simulink model "sampleModel1987"  (R2023a)
settings: Solver=VariableStepAuto  StartTime=0.0  StopTime=10.0  RelTol=1e-3
libraries: hdlsllib x4, simulink x3
settings Model: Creator=user1  LastModifiedBy=user1

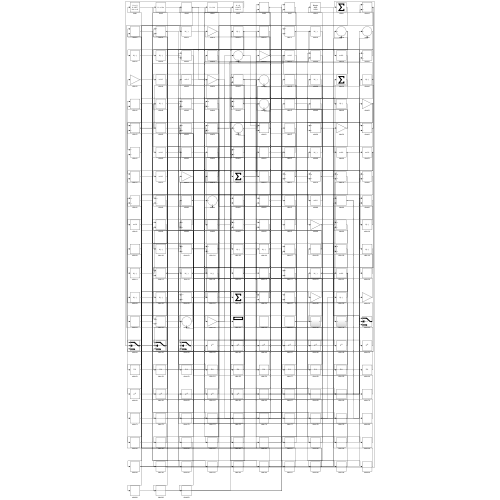
[thumbnail: Simulink's stored preview of the top-level diagram]
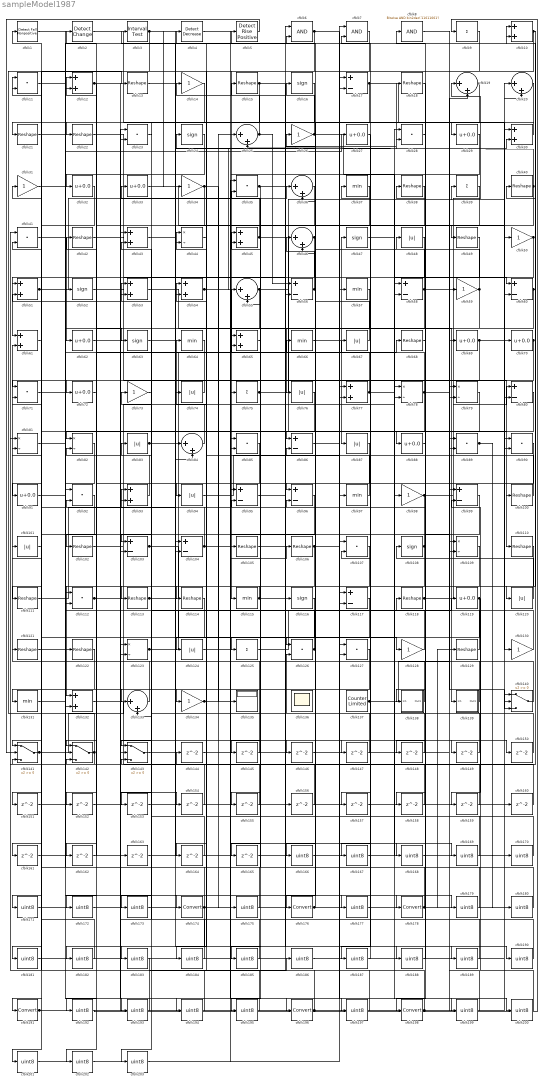
== system sampleModel1987 ==
  cfblk1 : hdlsllib/Logic and Bit Operations/Detect Fall Nonpositive  vinit=0  OutDataTypeStr=boolean
  cfblk{10,12,30,43,45,51,53..54,61,65,77,93,132} (13 alike) : Sum
  cfblk{13,15,18,21..22,38,40,42,49,68,100,102,105..106,110..111,113..114,118,121..122,129} (22 alike) : Reshape
  cfblk{48,67,74,76,83,87,94,101,120,124} (10 alike) : Abs  SaturateOnIntegerOverflow=off
  cfblk{17,56,58,60,80,86,95..96,99,103..104,117} (12 alike) : Sum  Inputs=+-
  cfblk{11,23,28,35,41,71,85,89..90,92,107,112,126..127} (14 alike) : DotProduct  OutDataTypeStr=Inherit: Inherit via internal rule
  cfblk{16,24,47,52,63,108,116} (7 alike) : Signum
  cfblk{44,78..79,81..82,109,123} (7 alike) : Product  Inputs=*/  RndMeth=Zero  SaturateOnIntegerOverflow=on
  cfblk{37,57,64,66,97,115,131} (7 alike) : MinMax
  cfblk{27,29,32..33,62,69..70,72,88,91,119} (11 alike) : Bias  Bias=0.0  SaturateOnIntegerOverflow=off
  cfblk{9,39,75,125} (4 alike) : Sum  Inputs=+
  cfblk{14,26,31,34,50,59,73,98,128,130,134} (11 alike) : Gain
  cfblk{19..20,25,36,46,55,84,133} (8 alike) : Sum  Inputs=|++
  cfblk135 : Display
  cfblk136 : Scope
      settings: Floating=on
  cfblk137 : hdlsllib/Sources/Counter Limited  uplimit=7  tsamp=-1
  cfblk138 : Subsystem
      settings: LibrarySourceBlock=|
      | hdlsllib/Ports &
      | Subsystems/Subsystem
  cfblk139 : Subsystem
      settings: LibrarySourceBlock=|
      | hdlsllib/Ports &
      | Subsystems/Subsystem
  cfblk{140..143} (4 alike) : Switch  SaturateOnIntegerOverflow=off  InputSameDT=off
  cfblk{144..165} (22 alike) : Delay  SampleTime=1
  cfblk{166..173,175,177,179..190,192..195,197,199..203} (32 alike) : DataTypeConversion  OutDataTypeStr=uint8  SaturateOnIntegerOverflow=off  RndMeth=Floor
  cfblk{174,176,178,191,196,198} (6 alike) : DataTypeConversion  SaturateOnIntegerOverflow=off  RndMeth=Floor
  cfblk2 : simulink/Logic and Bit Operations/Detect Change  vinit=0  OutDataTypeStr=boolean
      settings: LibrarySourceBlock=|
      | hdlsllib/Logic and Bit
      | Operations/Detect
      | Change
  cfblk3 : hdlsllib/Logic and Bit Operations/Interval Test  IntervalClosedRight=on  uplimit=0.5  IntervalClosedLeft=on  lowlimit=-0.5  OutDataTypeStr=boolean
  cfblk4 : simulink/Logic and Bit Operations/Detect Decrease  vinit=0.0  OutDataTypeStr=boolean
      settings: LibrarySourceBlock=|
      | hdlsllib/Logic and Bit
      | Operations/Detect
      | Decrease
  cfblk5 : hdlsllib/Logic and Bit Operations/Detect Rise Positive  vinit=0  OutDataTypeStr=boolean
  cfblk6 : Logic  AllPortsSameDT=off  OutDataTypeStr=boolean
  cfblk7 : Logic  AllPortsSameDT=off  OutDataTypeStr=boolean
  cfblk8 : simulink/Logic and Bit Operations/Bitwise Operator  logicop=AND  UseBitMask=on  BitMask=bin2dec('11011001')  BitMaskRealWorld=Stored Integer
      settings: LibrarySourceBlock=|
      | hdlsllib/Logic and Bit
      | Operations/Bitwise
      | Operator
  wires:
  cfblk16/1 -> cfblk21/1
  cfblk17/1 -> cfblk29/1, cfblk46/2
  cfblk29/1 -> cfblk115/1
  cfblk54/1 -> cfblk18/1, cfblk149/1
  cfblk77/1 -> cfblk47/1, cfblk189/1
  cfblk46/1 -> cfblk61/1, cfblk65/2
  cfblk84/1 -> cfblk64/1
  cfblk118/1 -> cfblk19/1, cfblk140/3
  cfblk133/1 -> cfblk61/2
  cfblk61/1 -> cfblk11/1
  cfblk63/1 -> cfblk86/1
  cfblk66/1 -> cfblk87/1
  cfblk100/1 -> cfblk54/1
  cfblk7/1 -> cfblk75/1
  cfblk113/1 -> cfblk55/1, cfblk147/1
  cfblk51/1 -> cfblk36/1, cfblk27/1
  cfblk132/1 -> cfblk40/1
  cfblk35/1 -> cfblk125/1, cfblk79/2, cfblk190/1
  cfblk30/1 -> cfblk22/1
  cfblk86/1 -> cfblk97/1
  cfblk95/1 -> cfblk178/1
  cfblk121/1 -> cfblk174/1
  cfblk68/1 -> cfblk38/1
  cfblk2/1 -> cfblk130/1
  cfblk110/1 -> cfblk132/1
  cfblk142/1 -> cfblk13/1, cfblk141/3
  cfblk55/1 -> cfblk39/1, cfblk124/1
  cfblk70/1 -> cfblk72/1, cfblk203/1
  cfblk75/1 -> cfblk20/1, cfblk28/2
  cfblk139/1(Out1) -> cfblk55/2
  cfblk103/1 -> cfblk128/1, cfblk30/2
  cfblk126/1 -> cfblk44/1, cfblk83/1
  cfblk141/1 -> cfblk28/1, cfblk119/1
  cfblk58/1 -> cfblk3/1, cfblk140/2, cfblk192/1
  cfblk41/1 -> cfblk62/1
  cfblk115/1 -> cfblk113/1, cfblk68/1
  cfblk22/1 -> cfblk135/1
  cfblk20/1 -> cfblk23/2
  cfblk93/1 -> cfblk12/1
  cfblk79/1 -> cfblk82/1
  cfblk83/1 -> cfblk53/1, cfblk5/1
  cfblk15/1 -> cfblk112/2, cfblk49/1, cfblk153/1
  cfblk87/1 -> cfblk133/1
  cfblk52/1 -> cfblk110/1
  cfblk104/1 -> cfblk2/1, cfblk134/1, cfblk197/1
  cfblk102/1 -> cfblk17/1
  cfblk62/1 -> cfblk98/1
  cfblk10/1 -> cfblk120/1, cfblk164/1
  cfblk80/1 -> cfblk111/1
  cfblk26/1 -> cfblk14/1, cfblk78/2
  cfblk42/1 -> cfblk116/1
  cfblk45/1 -> cfblk100/1, cfblk33/1
  cfblk78/1 -> cfblk131/1, cfblk42/1, cfblk19/2
  cfblk53/1 -> cfblk139/1(In1)
  cfblk72/1 -> cfblk12/2
  cfblk97/1 -> cfblk54/2
  cfblk109/1 -> cfblk143/1
  cfblk125/1 -> cfblk57/1
  cfblk48/1 -> cfblk85/2
  cfblk96/1 -> cfblk105/1
  cfblk82/1 -> cfblk132/2
  cfblk74/1 -> cfblk71/1
  cfblk23/1 -> cfblk103/1
  cfblk24/1 -> cfblk32/1
  cfblk1/1 -> cfblk109/2
  cfblk140/1 -> cfblk71/2
  cfblk44/1 -> cfblk94/1
  cfblk21/1 -> cfblk63/1
  cfblk13/1 -> cfblk126/1
  cfblk57/1 -> cfblk76/1
  cfblk65/1 -> cfblk45/1
  cfblk71/1 -> cfblk88/1
  cfblk50/1 -> cfblk58/2, cfblk187/1
  cfblk112/1 -> cfblk154/1, cfblk194/1
  cfblk8/1 -> cfblk69/1
  cfblk32/1 -> cfblk91/1
  cfblk138/1(Out1) -> cfblk93/1
  cfblk37/1 -> cfblk176/1
  cfblk11/1 -> cfblk103/2
  cfblk36/1 -> cfblk104/2
  cfblk19/1 -> cfblk52/1, cfblk102/1
  cfblk12/1 -> cfblk122/1, cfblk150/1
  cfblk114/1 -> cfblk141/1
  cfblk69/1 -> cfblk30/1, cfblk157/1
  cfblk134/1 -> cfblk106/1, cfblk25/1
  cfblk47/1 -> cfblk60/1
  cfblk5/1 -> cfblk141/2
  cfblk3/1 -> cfblk51/1, cfblk34/1, cfblk56/2
  cfblk120/1 -> cfblk108/1
  cfblk91/1 -> cfblk66/1
  cfblk137/1 -> cfblk59/1, cfblk200/1
  cfblk129/1 -> cfblk86/2
  cfblk31/1 -> cfblk196/1
  cfblk6/1 -> cfblk114/1, cfblk168/1
  cfblk89/1 -> cfblk170/1, cfblk180/1
  cfblk123/1 -> cfblk17/2, cfblk133/2
  cfblk119/1 -> cfblk138/1(In1), cfblk159/1, cfblk172/1
  cfblk9/1 -> cfblk191/1
  cfblk67/1 -> cfblk16/1
  cfblk33/1 -> cfblk70/1
  cfblk40/1 -> cfblk93/2, cfblk25/2
  cfblk88/1 -> cfblk8/1
  cfblk38/1 -> cfblk45/2
  cfblk59/1 -> cfblk24/1, cfblk112/1, cfblk7/2
  cfblk14/1 -> cfblk142/1
  cfblk128/1 -> cfblk65/1
  cfblk98/1 -> cfblk80/1, cfblk92/2
  cfblk94/1 -> cfblk77/1
  cfblk25/1 -> cfblk15/1, cfblk56/1
  cfblk99/1 -> cfblk198/1
  cfblk34/1 -> cfblk162/1, cfblk175/1
  cfblk56/1 -> cfblk46/1, cfblk96/1
  cfblk108/1 -> cfblk41/2, cfblk96/2, cfblk173/1
  cfblk131/1 -> cfblk10/1
  cfblk111/1 -> cfblk84/2
  cfblk60/1 -> cfblk10/2, cfblk195/1
  cfblk130/1 -> cfblk53/2
  cfblk106/1 -> cfblk123/2, cfblk199/1
  cfblk144/1 -> cfblk109/1
  cfblk39/1 -> cfblk145/1
  cfblk145/1 -> cfblk1/1
  cfblk124/1 -> cfblk146/1
  cfblk146/1 -> cfblk77/2
  cfblk147/1 -> cfblk51/2
  cfblk18/1 -> cfblk148/1
  cfblk148/1 -> cfblk104/1
  cfblk149/1 -> cfblk36/2
  cfblk150/1 -> cfblk126/2
  cfblk122/1 -> cfblk151/1
  cfblk151/1 -> cfblk123/1
  cfblk85/1 -> cfblk152/1
  cfblk152/1 -> cfblk84/1
  cfblk153/1 -> cfblk58/1
  cfblk154/1 -> cfblk82/2
  cfblk49/1 -> cfblk155/1
  cfblk155/1 -> cfblk143/2
  cfblk105/1 -> cfblk156/1
  cfblk156/1 -> cfblk35/2
  cfblk157/1 -> cfblk80/2
  cfblk28/1 -> cfblk158/1
  cfblk158/1 -> cfblk41/1
  cfblk159/1 -> cfblk6/2
  cfblk160/1 -> cfblk142/2
  cfblk92/1 -> cfblk161/1
  cfblk161/1 -> cfblk60/2
  cfblk162/1 -> cfblk142/3
  cfblk163/1 -> cfblk44/2
  cfblk164/1 -> cfblk143/3
  cfblk116/1 -> cfblk165/1
  cfblk165/1 -> cfblk78/1
  cfblk90/1 -> cfblk166/1
  cfblk166/1 -> cfblk67/1
  cfblk27/1 -> cfblk167/1
  cfblk167/1 -> cfblk90/1
  cfblk168/1 -> cfblk90/2
  cfblk4/1 -> cfblk169/1
  cfblk169/1 -> cfblk48/1
  cfblk170/1 -> cfblk4/1
  cfblk127/1 -> cfblk171/1
  cfblk171/1 -> cfblk20/2
  cfblk172/1 -> cfblk127/1
  cfblk173/1 -> cfblk127/2
  cfblk174/1 -> cfblk92/1, cfblk179/1, cfblk202/1
  cfblk175/1 -> cfblk121/1
  cfblk176/1 -> cfblk79/1, cfblk26/1
  cfblk143/1 -> cfblk177/1
  cfblk177/1 -> cfblk37/1
  cfblk178/1 -> cfblk140/1, cfblk129/1, cfblk23/1
  cfblk179/1 -> cfblk95/1
  cfblk180/1 -> cfblk95/2
  cfblk101/1 -> cfblk181/1
  cfblk181/1 -> cfblk50/1
  cfblk64/1 -> cfblk182/1
  cfblk182/1 -> cfblk101/1
  cfblk73/1 -> cfblk183/1
  cfblk76/1 -> cfblk184/1
  cfblk184/1 -> cfblk73/1
  cfblk107/1 -> cfblk185/1
  cfblk185/1 -> cfblk144/1
  cfblk183/1 -> cfblk186/1
  cfblk186/1 -> cfblk107/1
  cfblk187/1 -> cfblk107/2
  cfblk43/1 -> cfblk188/1
  cfblk188/1 -> cfblk118/1
  cfblk189/1 -> cfblk43/1
  cfblk190/1 -> cfblk43/2
  cfblk191/1 -> cfblk163/1, cfblk89/2, cfblk7/1
  cfblk192/1 -> cfblk9/1
  cfblk81/1 -> cfblk193/1
  cfblk193/1 -> cfblk11/2
  cfblk194/1 -> cfblk81/1
  cfblk195/1 -> cfblk81/2
  cfblk196/1 -> cfblk89/1, cfblk74/1
  cfblk197/1 -> cfblk31/1
  cfblk198/1 -> cfblk160/1, cfblk6/1, cfblk35/1
  cfblk199/1 -> cfblk99/1
  cfblk200/1 -> cfblk99/2
  cfblk117/1 -> cfblk201/1
  cfblk201/1 -> cfblk85/1
  cfblk202/1 -> cfblk117/1
  cfblk203/1 -> cfblk117/2

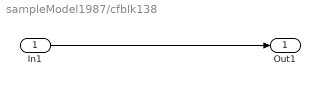
== system sampleModel1987/cfblk138 ==
  In1 : Inport
  Out1 : Outport
  wires:
  In1/1 -> Out1/1

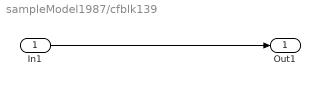
== system sampleModel1987/cfblk139 ==
  In1 : Inport
  Out1 : Outport
  wires:
  In1/1 -> Out1/1
